simulink model "Es1"  (R2014a)
settings: Solver=ode45  StartTime=0.0  StopTime=100  RelTol=1e-3
values from neighbouring files (symbols this model uses):
  s = tf('s')    [Es1.m]
libraries: cstblocks x4, simulink x1
settings Model: Creator=Davide  LastModifiedBy=Davide

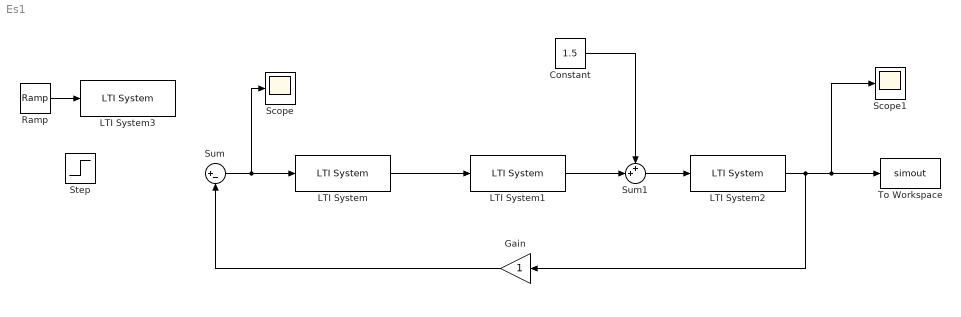
== system Es1 ==
  Constant : Constant  Value=1.5
  Gain : Gain
  LTI System : cstblocks/LTI System  sys=C  IC=[]
  LTI System1 : cstblocks/LTI System  sys=F1  IC=[]
  LTI System2 : cstblocks/LTI System  sys=F2  IC=[]
  LTI System3 : cstblocks/LTI System  sys=1/s  IC=[]
  Ramp : simulink/Sources/Ramp  slope=1  start=0  X0=0
  Scope : Scope
  Scope1 : Scope
  Step : Step  SampleTime=0
  Sum : Sum  Inputs=|+-
  Sum1 : Sum  Inputs=++|
  To Workspace : ToWorkspace  VariableName=simout  SaveFormat=Timeseries  SampleTime=-1
  wires:
  LTI System/1 -> LTI System1/1
  LTI System1/1 -> Sum1/2
  Sum1/1 -> LTI System2/1
  Gain/1 -> Sum/2
  Sum/1 -> Scope/1, LTI System/1
  LTI System2/1 -> Gain/1, Scope1/1, To Workspace/1
  Ramp/1 -> LTI System3/1
  Constant/1 -> Sum1/1
